simulink model "dc_motor_model_for_3dsim_by_Tejas"  (R2019b)
settings: Solver=VariableStepAuto  StartTime=0.0  StopTime=10.0  RelTol=1e-3
libraries: fl_lib x7, nesl_utility x4, ee_lib x1, sm_lib x1
settings Model: Creator=RAJENDRA PHUTANE  LastModifiedBy=RAJENDRA PHUTANE

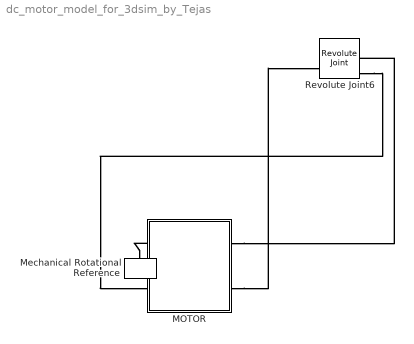
== system dc_motor_model_for_3dsim_by_Tejas ==
  MOTOR : Subsystem
  Mechanical Rotational Reference : fl_lib/Mechanical/Rotational Elements/Mechanical Rotational Reference
  Revolute Joint6 : sm_lib/Joints/Revolute Joint  JointMode=Normal  SenseConstraintForce=off  SenseConstraintForceX=off  SenseConstraintForceY=off  SenseConstraintForceZ=off  SenseConstraintTorque=off  SenseConstraintTorqueX=off  SenseConstraintTorqueY=off  SenseConstraintTorqueZ=off  SenseTotalForce=off  SenseTotalForceX=off  SenseTotalForceY=off  SenseTotalForceZ=off  SenseTotalTorque=off  SenseTotalTorqueX=off  SenseTotalTorqueY=off  SenseTotalTorqueZ=off  CompositeWrenchDir=BaseOnFollower  CompositeWrenchFrame=BaseFrame  EquilibriumPosition=0  EquilibriumPositionUnits=deg  SpringStiffness=0  SpringStiffnessUnits=N*m/deg  DampingCoefficient=0  DampingCoefficientUnits=N*m/(deg/s)  TorqueActuationMode=InputTorque  MotionActuationMode=ComputedMotion  SensePosition=off  SenseVelocity=on  SenseAcceleration=off  SenseTorqueForce=on  SenseLowerLimitTorqueForce=off  SenseUpperLimitTorqueForce=off  LowerLimitSpecify=on  LowerLimitBound=-1.5  LowerLimitBoundUnits=deg  LowerLimitStiffness=1e4  LowerLimitStiffnessUnits=N*m/deg  LowerLimitDamping=10  LowerLimitDampingUnits=N*m/(deg/s)  LowerLimitTransitionRegionWidth=0.1  LowerLimitTransitionRegionWidthUnits=deg  UpperLimitSpecify=on  UpperLimitBound=40  UpperLimitBoundUnits=deg  UpperLimitStiffness=1e4  UpperLimitStiffnessUnits=N*m/deg  UpperLimitDamping=10  UpperLimitDampingUnits=N*m/(deg/s)  UpperLimitTransitionRegionWidth=0.1  UpperLimitTransitionRegionWidthUnits=deg  PositionTargetSpecify=off  PositionTargetPriority=High  PositionTargetValue=0  PositionTargetValueUnits=deg  VelocityTargetSpecify=on  VelocityTargetPriority=High  VelocityTargetValue=3  VelocityTargetValueUnits=rev/s
  connections:
  MOTOR/LConn1 -- Mechanical Rotational Reference/LConn1
  Revolute Joint6/RConn3 -- MOTOR/LConn2
  MOTOR/RConn1 -- Revolute Joint6/RConn2
  MOTOR/RConn2 -- Revolute Joint6/LConn2

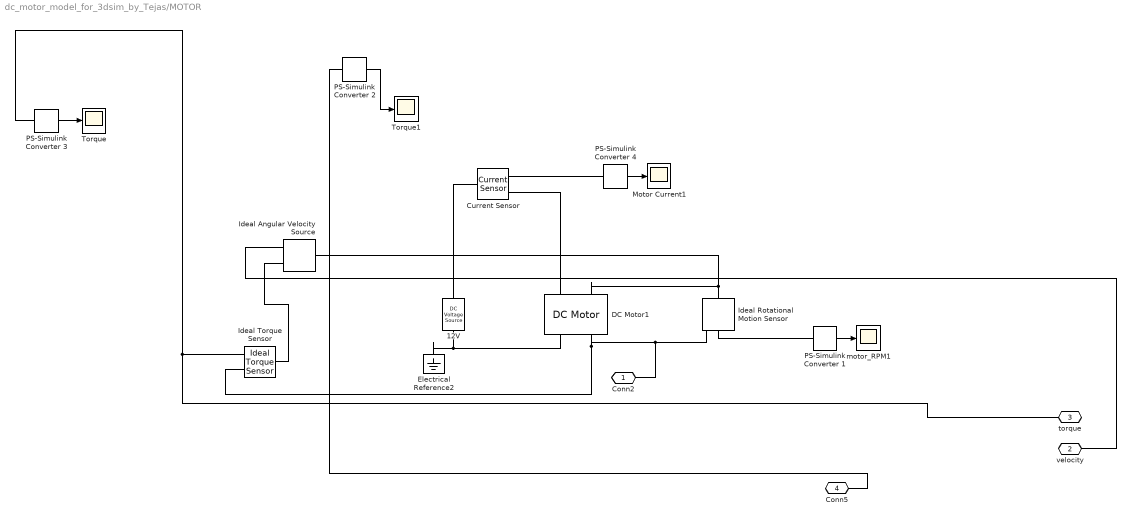
== system dc_motor_model_for_3dsim_by_Tejas/MOTOR ==
  12V : fl_lib/Electrical/Electrical Sources/DC Voltage Source  v0=18 V
  Current Sensor : fl_lib/Electrical/Electrical Sensors/Current Sensor
  DC Motor1 : ee_lib/Electromechanical/Brushed Motors/DC Motor  parameterization=2  Ra=3.9 Ohm  La=0.01 H  emf_or_torque=1  Kv=0.072e-3 V/rpm  Ki=6.876e-4 N*m/A  T_stall=3.5 N*m  w_max=200 rpm  w_rated=15000 rpm  P_rated=0.08 W  V_rated=18 V  J=0.01 g*cm^2  lam_param=1  lam=0 N*m/(rad/s)  i_noload=2.7 A  V_i_noload=18 V  speed0=0 rpm  alpha=3.93e-3 1/K  Tmeas=25 degC  thermal_mass=100 J/K  initial_temperature=25 degC
      settings: SourceProductName=Simscape Electrical
  Electrical Reference2 : fl_lib/Electrical/Electrical Elements/Electrical Reference
  Ideal Angular Velocity Source : fl_lib/Mechanical/Mechanical Sources/Ideal Angular Velocity Source
  Ideal Rotational Motion Sensor : fl_lib/Mechanical/Mechanical Sensors/Ideal Rotational Motion Sensor  offset=0 rad
  Ideal Torque Sensor : fl_lib/Mechanical/Mechanical Sensors/Ideal Torque Sensor
  Motor Current1 : Scope
  PS-Simulink Converter 1 : nesl_utility/PS-Simulink Converter  PhysicalDomain=network_engine_domain  SubClassName=ps_output  LeftPortType=input  RightPortType=output  PseudoPeriodic=off  Frequencies=[]  Unit=rpm  AffineConversion=off
  PS-Simulink Converter 2 : nesl_utility/PS-Simulink Converter  PhysicalDomain=network_engine_domain  SubClassName=ps_output  LeftPortType=input  RightPortType=output  PseudoPeriodic=off  Frequencies=[]  Unit=N*m  AffineConversion=off
  PS-Simulink Converter 3 : nesl_utility/PS-Simulink Converter  PhysicalDomain=network_engine_domain  SubClassName=ps_output  LeftPortType=input  RightPortType=output  PseudoPeriodic=off  Frequencies=[]  Unit=N*m  AffineConversion=off
  PS-Simulink Converter 4 : nesl_utility/PS-Simulink Converter  PhysicalDomain=network_engine_domain  SubClassName=ps_output  LeftPortType=input  RightPortType=output  PseudoPeriodic=off  Frequencies=[]  Unit=A  AffineConversion=off
  Torque : Scope
  Torque1 : Scope
  motor_RPM1 : Scope
  Conn2 : PMIOPort  Side=Left
  velocity : PMIOPort  Port=2  Side=Right
  torque : PMIOPort  Port=3  Side=Right
  Conn5 : PMIOPort  Port=4  Side=Left
  wires:
  PS-Simulink Converter 3/1 -> Torque/1
  PS-Simulink Converter 2/1 -> Torque1/1
  PS-Simulink Converter 1/1 -> motor_RPM1/1
  PS-Simulink Converter 4/1 -> Motor Current1/1
  connections:
  DC Motor1/LConn2 -- Ideal Rotational Motion Sensor/LConn1 -- Ideal Angular Velocity Source/LConn1
  DC Motor1/LConn1 -- Current Sensor/RConn2
  Ideal Torque Sensor/RConn1 -- Conn2/RConn1 -- Ideal Rotational Motion Sensor/RConn1 -- DC Motor1/RConn2
  DC Motor1/RConn1 -- Electrical Reference2/LConn1 -- 12V/RConn1
  Ideal Torque Sensor/LConn1 -- Ideal Angular Velocity Source/RConn2
  PS-Simulink Converter 3/LConn1 -- torque/RConn1 -- Ideal Torque Sensor/RConn2
  Current Sensor/RConn1 -- PS-Simulink Converter 4/LConn1
  12V/LConn1 -- Current Sensor/LConn1
  PS-Simulink Converter 1/LConn1 -- Ideal Rotational Motion Sensor/RConn2
  Conn5/RConn1 -- PS-Simulink Converter 2/LConn1
  Ideal Angular Velocity Source/RConn1 -- velocity/RConn1
